simulink model "Subsystem"  (R2020b)
settings: Solver=VariableStepAuto  StartTime=0.0  StopTime=10.0  RelTol=1e-3
undefined symbols (not defined in the file): b, m
settings Model: Creator=Pulkit Khandelwal  LastModifiedBy=Pulkit Khandelwal
settings DataIOCC: SaveOutput=off  SaveTime=off

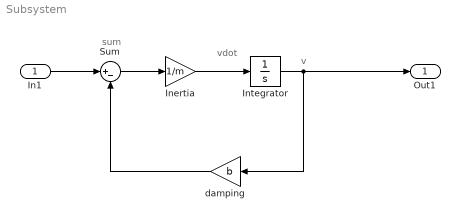
== system Subsystem ==
  note: v
  note: sum
  note: vdot
  In1 : Inport  OutDataTypeStr=single  PortDimensions=[1 1]  SampleTime=0
  Inertia : Gain  Gain=1/m
  Integrator : Integrator
  Sum : Sum  Inputs=|+-
  damping : Gain  Gain=b
  Out1 : Outport  OutDataTypeStr=double  PortDimensions=1  SampleTime=0
  wires:
  In1/1 -> Sum/1
  Integrator/1 -> damping/1, Out1/1
  Inertia/1 -> Integrator/1
  damping/1 -> Sum/2
  Sum/1 -> Inertia/1
